simulink model "Simulink"  (R2021a)
settings: Solver=ode4  StartTime=0.0  StopTime=10.0  FixedStep=0.0001  RelTol=1e-3
libraries: cstblocks x1
settings Model: Creator=Santiago  LastModifiedBy=Santiago

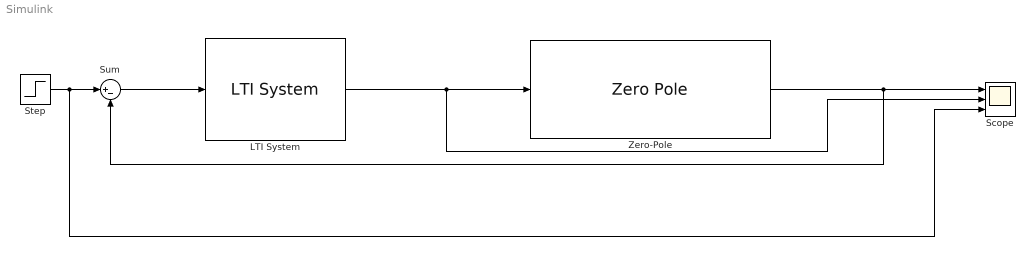
== system Simulink ==
  LTI System : cstblocks/LTI System  sys=C_digi  IC=[]
  Scope : Scope  NumInputPorts=3
  Step : Step  SampleTime=0
  Sum : Sum  Inputs=|+-
  Zero-Pole : ZeroPole  Zeros=[50]  Poles=[1/2, -50]  Gain=[-1]
  wires:
  LTI System/1 -> Scope/2, Zero-Pole/1
  Sum/1 -> LTI System/1
  Zero-Pole/1 -> Sum/2, Scope/1
  Step/1 -> Scope/3, Sum/1
